simulink model "sim_chua_fl_2012"  (Simulink 9.0)
settings: Solver=ode4  StartTime=0.0  StopTime=tfin  FixedStep=0.1  RelTol=1e-3
values from neighbouring files (symbols this model uses):
  C = [1 0 0]    [main_chua_fl.m]
  x0 = randn(3,1)*0    [main_chua_fl.m]
undefined symbols (not defined in the file or in its folder): fg_chua, u_chua
libraries: cstblocks x1
settings Model: SuppressorTable=22 serialization::archive 11 0 6 0 0 0 0 0  Creator=carlonovara  LastModifiedBy=carlonovara
settings DataIOCC: SaveFormat=StructureWithTime
settings DebuggingCC: UnderspecifiedInitializationDetection=Simplified  MergeDetectMultiDrivingBlocksExec=error  SFUnexpectedBacktrackingDiag=error  SFNoUnconditionalDefaultTransitionDiag=error
settings HardwareCC: ProdBitPerPointer=64  ProdLargestAtomicFloat=Float  ProdIntDivRoundTo=Zero  ProdEndianess=LittleEndian  ProdHWDeviceType=Specified
settings ModelReferenceCC: PropagateSignalLabelsOutOfModel=on
settings GRTTargetCC: TargetLangStandard=C99 (ISO)
settings ConfigComp: CovMetricSettings=dwe  CovHtmlReporting=off  CovSaveCumulativeToWorkspaceVar=off  CovSaveSingleToWorkspaceVar=off  CovExternalEMLEnable=on

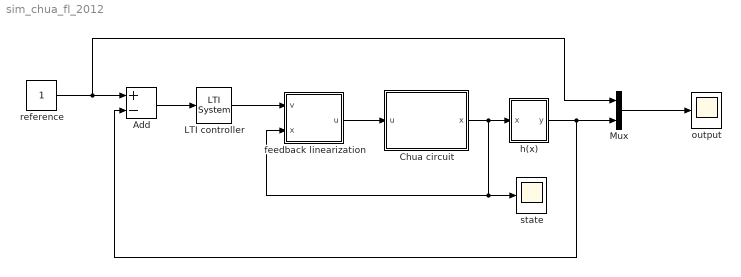
== system sim_chua_fl_2012 ==
  Add : Sum  Inputs=+-
  Chua circuit : Subsystem
  LTI controller : cstblocks/LTI System  sys=K  IC=[]
  Mux : Mux  Inputs=2
  feedback linearization : Subsystem
  h(x) : Subsystem
  output : Scope
  reference : Constant
  state : Scope
  wires:
  Chua circuit/1(x) -> h(x)/1(x), state/1, feedback linearization/2(x)
  feedback linearization/1(u) -> Chua circuit/1(u)
  h(x)/1(y) -> Add/2, Mux/2
  Add/1 -> LTI controller/1
  LTI controller/1 -> feedback linearization/1(v)
  Mux/1 -> output/1
  reference/1 -> Mux/1, Add/1

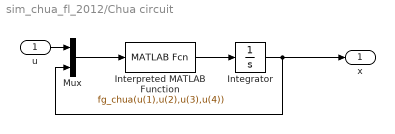
== system sim_chua_fl_2012/Chua circuit ==
  u : Inport
  Integrator : Integrator  InitialCondition=x0
  Interpreted MATLAB Function : MATLABFcn  MATLABFcn=fg_chua(u(1),u(2),u(3),u(4))  OutputDimensions=3
  Mux : Mux  Inputs=2
  x : Outport
  wires:
  u/1 -> Mux/1
  Interpreted MATLAB Function/1 -> Integrator/1
  Integrator/1 -> Mux/2, x/1
  Mux/1 -> Interpreted MATLAB Function/1

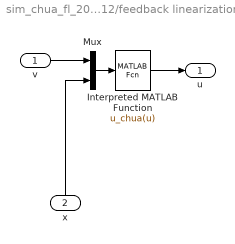
== system sim_chua_fl_2012/feedback linearization ==
  v : Inport
  x : Inport  Port=2
  Interpreted MATLAB Function : MATLABFcn  MATLABFcn=u_chua(u)
  Mux : Mux  Inputs=2
  u : Outport
  wires:
  x/1 -> Mux/2
  Mux/1 -> Interpreted MATLAB Function/1
  Interpreted MATLAB Function/1 -> u/1
  v/1 -> Mux/1

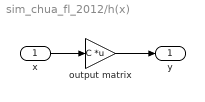
== system sim_chua_fl_2012/h(x) ==
  x : Inport
  output matrix : Gain  Gain=C  Multiplication=Matrix(K*u)
  y : Outport
  wires:
  x/1 -> output matrix/1
  output matrix/1 -> y/1
